simulink model "Combined"  (R2023b)
settings: Solver=VariableStepAuto  StartTime=0.0  StopTime=10.0  RelTol=1e-3
undefined symbols (not defined in the file or in its folder): a, B1, B2, Bc, J1, J2, Jc
settings Model: Creator=joshc  LastModifiedBy=joshc

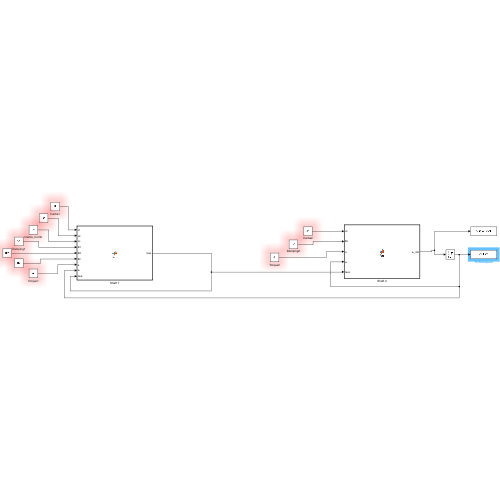
[thumbnail: Simulink's stored preview of the top-level diagram]
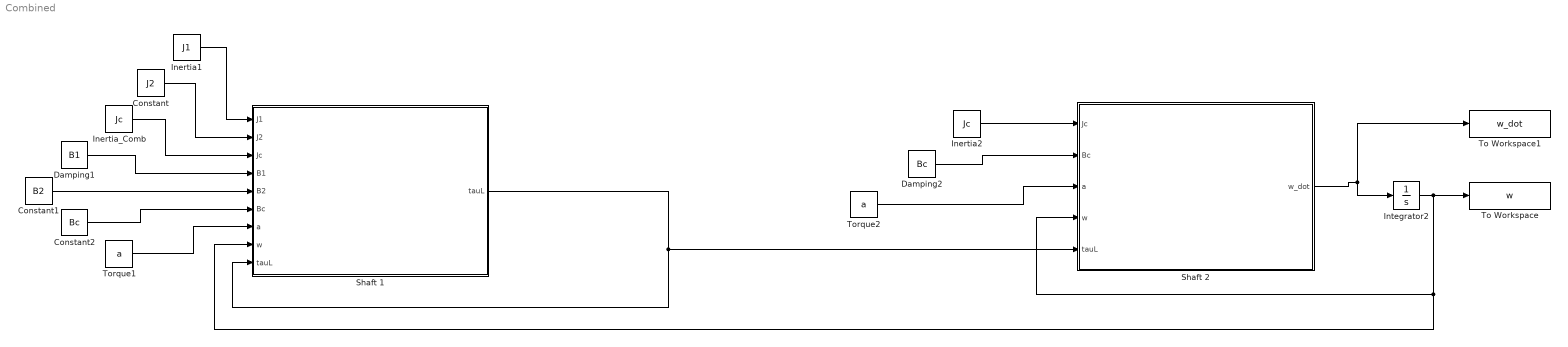
== system Combined ==
  Constant : Constant  Value=J2
  Constant1 : Constant  Value=B2
  Constant2 : Constant  Value=Bc
  Damping1 : Constant  Value=B1
  Damping2 : Constant  Value=Bc
  Inertia1 : Constant  Value=J1
  Inertia2 : Constant  Value=Jc
  Inertia_Comb : Constant  Value=Jc
  Integrator2 : Integrator  LimitOutput=on  UpperSaturationLimit=1000
  Shaft 1 : MATLAB Function  TreatAsAtomicUnit=on
  Shaft 2 : MATLAB Function  TreatAsAtomicUnit=on
  To Workspace : ToWorkspace  VariableName=w  SaveFormat=Timeseries  SampleTime=-1
  To Workspace1 : ToWorkspace  VariableName=w_dot  SaveFormat=Structure With Time  SampleTime=-1
  Torque1 : Constant  Value=a
  Torque2 : Constant  Value=a
  wires:
  Torque1/1 -> Shaft 1/7(a)
  Inertia1/1 -> Shaft 1/1(J1)
  Damping1/1 -> Shaft 1/4(B1)
  Integrator2/1 -> Shaft 1/8(w), Shaft 2/4(w), To Workspace/1
  Shaft 2/1(w_dot) -> To Workspace1/1, Integrator2/1
  Torque2/1 -> Shaft 2/3(a)
  Damping2/1 -> Shaft 2/2(Bc)
  Inertia2/1 -> Shaft 2/1(Jc)
  Constant/1 -> Shaft 1/2(J2)
  Inertia_Comb/1 -> Shaft 1/3(Jc)
  Constant1/1 -> Shaft 1/5(B2)
  Constant2/1 -> Shaft 1/6(Bc)
  Shaft 1/1(tauL) -> Shaft 1/9("tauL "), Shaft 2/5(tauL)

== matlab function Combined/Shaft 1 ==
  data: J1 input; J2 input; Jc input; tauL output; B1 input; B2 input; Bc input; a input; w input; tauL input
function tauL = fcn(J1, J2, Jc, B1, B2, Bc, a, w, tauL)

tauL = ((1/Jc)*(J2*a + J2*tauL)) - ((1/Jc)*(B1*J2 - B2*J1)*w);

end

== matlab function Combined/Shaft 2 ==
  data: Jc input; w_dot output; Bc input; a input; w input; tauL input
function w_dot = fcn(Jc, Bc, a, w, tauL)

w_dot = ((1/Jc)*(a - tauL)) - ((Bc/Jc)*w);

end
